simulink model "entreg2"  (R2019a)
settings: Solver=ode4  StartTime=0.0  StopTime=148  FixedStep=0.04  RelTol=1e-3
undefined symbols (not defined in the file or in its folder): Angular, Linear
libraries: robotlib x4, simulink x2, fuzblock x1
settings Model: Creator=LMI-01  LastModifiedBy=lucas
settings DataIOCC: ReturnWorkspaceOutputs=off
settings DebuggingCC: PregeneratedLibrarySubsystemCodeDiagnostic=none  ArithmeticOperatorsInVariantConditions=warning
settings SFSimCC: SimUseLocalCustomCode=off
settings RTWCC: RTWUseLocalCustomCode=off

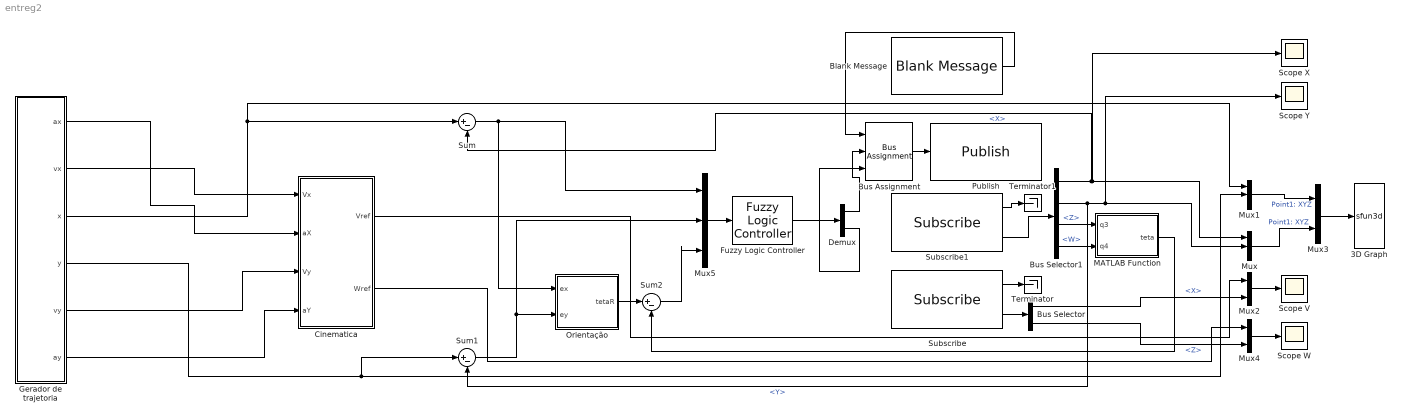
== system entreg2 ==
  3D Graph : S-Function  LoadFcn=if exist('sfun3d','file'), sfun3d([],[],[],'LoadBlock'); end  FunctionName=sfun3d  Parameters=ax,T,np,cp,gd,ls,mk,mx,hd,tb  SFunctionDeploymentMode=off  EnableBusSupport=off  mask(3D Graph){np=2, ax=[-6 6 -6 6 -3 3], mx=1e4, T=0.04, cp=[0 0 1], gd=on, hd=off, tb=on, ls=-, mk=none}
      mask prompts: np "Number of moving points (lines)"; ax "Range: [xmin xmax  ymin ymax zmin zmax]"; mx "Max number of points in each line"; T "Sampling Time"; cp "Camera position (use [0 0 1] for 2D XY view)"; gd "Grid (on|off)"; hd "HeadMarkers (on|off)"; tb "Toolbar (on|off)"; ls "LineStyle"; mk "LineMarker"
      mask help:
      | This block plots the position of several points in the XYZ space. The input contains the coordinates of all the points (x1,y1,z1,x2,y2,z2,...).
      | The number of moving points (lines), the XYZ ranges, sampling time, camera position, and grid (among other things) can be set as mask parameters.
      settings: CopyFcn=if exist('sfun3d','file'), sfun3d([],[],[],'CopyBlock'); end  DeleteFcn=if exist('sfun3d','file'), sfun3d([],[],[],'DeleteBlock'); end  NameChangeFcn=if exist('sfun3d','file'), sfun3d([],[],[],'NameChange'); end
      mask Help:
      | This block plots the position of several points in the XYZ space. The input contains the coordinates of all the points (x1,y1,z1,x2,y2,z2,...).
      | The number of moving points (lines), the XYZ ranges, sampling time, camera position, and grid (among other things) can be set as mask parameters.
      mask TypeOptions ls: - | -- | : | -. | none
      mask TypeOptions mk: none | . | + | o | * | x | square | diamond | v | ^ | > | < | pentagram | hexagram
      mask Display: plot([.05 .95 .95 .05 .05],[.45 .45 .95 .95 .45], 0.5+cos(0:0.1:2*pi)*0.3,0.7+sin(0:0.1:2*pi)*0.2)
  Blank Message : robotlib/Blank Message  messageClass=Message  entityType=geometry_msgs/Twist  messageType=geometry_msgs/Twist  SampleTime=inf
      settings: SourceProductBaseCode=RO
  Bus Assignment : BusAssignment  AssignedSignals=Linear.X,Angular.Z
  Bus Selector : BusSelector  OutputSignals=Linear.X,Angular.Z
  Bus Selector1 : BusSelector  OutputSignals=Pose.Pose.Position.X,Pose.Pose.Position.Y,Pose.Pose.Orientation.Z,Pose.Pose.Orientation.W
  Cinematica : MATLAB Function  TreatAsAtomicUnit=on
  Demux : Demux  Outputs=2
  Fuzzy Logic Controller : fuzblock/Fuzzy Logic  Controller  FIS='controlador_fuzzy2.fis'  OutputSampleNumber=101  DataType=double  FuzzifiedInputs=off  RuleFiringStrengths=off  RuleOutputs=off  AggregatedOutputs=off  SimulateUsing=Interpreted execution  OutOfRangeInputValueMessage=warning  NoRuleFiredMessage=warning  EmptyOutputFuzzySetMessage=warning
  "Gerador de trajetoria " : Subsystem
  MATLAB Function : MATLAB Function  TreatAsAtomicUnit=on
  Mux : Mux  Inputs=3
  Mux1 : Mux  Inputs=3
  Mux2 : Mux  Inputs=2
  Mux3 : Mux  Inputs=2
  Mux4 : Mux  Inputs=2
  Mux5 : Mux  Inputs=3
  Orientação : MATLAB Function  TreatAsAtomicUnit=on
  Publish : robotlib/Publish  topicSource=Select from ROS network  topic=/mobile_base/commands/velocity  messageType=geometry_msgs/Twist  messageQueueLength=1
      settings: SourceProductBaseCode=RO
  Scope V : Scope
  Scope W : Scope
  Scope X : Scope
  Scope Y : Scope
  Subscribe : robotlib/Subscribe  topicSource=Select from ROS network  topic=/mobile_base/commands/velocity  messageType=geometry_msgs/Twist  sampleTime=-1  messageQueueLength=1
      settings: SourceProductBaseCode=RO
  Subscribe1 : robotlib/Subscribe  topicSource=Select from ROS network  topic=/odom  messageType=nav_msgs/Odometry  sampleTime=-1  messageQueueLength=1
      settings: SourceProductBaseCode=RO
  Sum : Sum  Inputs=|+-
  Sum1 : Sum  Inputs=|+-
  Sum2 : Sum  Inputs=|+-
  Terminator : Terminator
  Terminator1 : Terminator
  wires:
  Mux/1 -> Mux3/2  "Point1: XYZ"
  Mux1/1 -> Mux3/1  "Point1: XYZ"
  Mux3/1 -> 3D Graph/1
  Bus Assignment/1 -> Publish/1
  Subscribe1/1 -> Terminator1/1
  Subscribe/1 -> Terminator/1
  Subscribe1/2 -> Bus Selector1/1
  Subscribe/2 -> Bus Selector/1
  Mux2/1 -> Scope V/1
  Mux4/1 -> Scope W/1
  Bus Selector1/4 -> MATLAB Function/2(q4)  "<W>"
  Bus Selector1/3 -> MATLAB Function/1(q3)  "<Z>"
  Bus Selector1/1 -> Sum/2, Mux/1, Scope X/1  "<X>"
  Bus Selector1/2 -> Sum1/2, Mux/2, Scope Y/1  "<Y>"
  Bus Selector/2 -> Mux4/2  "<Z>"
  Bus Selector/1 -> Mux2/2  "<X>"
  "Gerador de trajetoria "/6(ay) -> Cinematica/4(aY)
  "Gerador de trajetoria "/1(ax) -> Cinematica/2(aX)
  Cinematica/1(Vref) -> Mux2/1
  Sum2/1 -> Mux5/3
  Orientação/1(tetaR) -> Sum2/1
  Fuzzy Logic Controller/1 -> Demux/1
  Sum/1 -> Orientação/1(ex), Mux5/1
  Sum1/1 -> Orientação/2(ey), Mux5/2
  MATLAB Function/1(teta) -> Sum2/2
  "Gerador de trajetoria "/2(vx) -> Cinematica/1(Vx)
  Demux/2 -> Bus Assignment/3
  Demux/1 -> Bus Assignment/2
  Cinematica/2(Wref) -> Mux4/1
  "Gerador de trajetoria "/5(vy) -> Cinematica/3(Vy)
  Mux5/1 -> Fuzzy Logic Controller/1
  Blank Message/1 -> Bus Assignment/1
  "Gerador de trajetoria "/3(x) -> Mux1/1, Sum/1
  "Gerador de trajetoria "/4(y) -> Mux1/2, Sum1/1

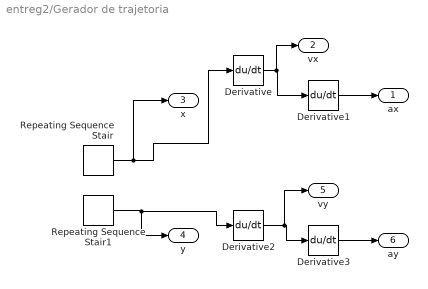
== system entreg2/Gerador de trajetoria  ==
  Derivative{,1..3} (4 alike) : Derivative
  Repeating Sequence Stair : simulink/Sources/Repeating Sequence Stair  OutValues=[0 0.35 0.7 1 1.17000000000000 1.13636630888818 1.29781681365468 1.46855831091587 1.63011117391398 1.86615524675713 2.01293235197162 2.16746647889735 2.18509923467053 2.19795065796801 2.19797948716949 2.22496970011073 2.24304671068726 2.23929618970334 2.26982794069553 2.26080362632337 2.38874656381839 2.50687255452925 2.60796600466398 2.75842470931807 2.91812309896753 3.09994531392603 3.21130779193203 3.37786059481534 3.37640575264878 3.45327720396131 3.47739985849164 3.52177306258873 3.57218392139281 3.68133849097106 3.84273878303952 3.97251349229218 4.19159254394481 4.39520776047253 4.72269852816546 5.06130600308634 5.36152509053121 5.59879385999157 5.61395180134724 5.57505150961989 5.56764716952759 5.51257506819779 5.51874953704695 5.50000000000000]  tsamp=3.20  OutMin=[]  OutMax=[]  OutDataTypeStr=double  OutputDataTypeScalingMode=double  OutDataType=fixdt(0,8)  ConRadixGroup=Best Precision: Vector-wise  OutScaling=2^-12
  Repeating Sequence Stair1 : simulink/Sources/Repeating Sequence Stair  OutValues=[-0.35 -0.35 -0.35 -0.35 0.0651893966525788 0.362129707732075 0.623753677382057 0.775354419626675 0.961745396579764 1.09086894927094 1.33822349520960 1.61879248910219 1.69784845568527 2.02858237206169 2.25979192143125 2.45253391279033 2.67050764424766 2.97554368142654 3.25003618292319 3.50994458764924 3.58083763030385 3.60607486682255 3.63371834792494 3.62325351902815 3.57869462970668 3.52263302654614 3.23603577016277 2.97281325291245 2.66960102131579 2.50992729488802 2.16798337821201 1.84910828582459 1.64510890890260 1.46272820883164 1.23525461377249 0.982385103207933 0.878102802302353 0.892639115809230 0.881338079577862 0.868529585350037 1.10708558244037 1.37592837094794 1.68515277057135 1.96863003655324 2.28149720632578 2.48742341640947 2.50000000000000]  tsamp=3.20  OutMin=[]  OutMax=[]  OutDataTypeStr=double  OutputDataTypeScalingMode=double  OutDataType=fixdt(0,8)  ConRadixGroup=Best Precision: Vector-wise  OutScaling=2^-12
  ax : Outport
  vx : Outport  Port=2
  x : Outport  Port=3
  y : Outport  Port=4
  vy : Outport  Port=5
  ay : Outport  Port=6
  wires:
  Derivative1/1 -> ax/1
  Derivative/1 -> vx/1, Derivative1/1
  Repeating Sequence Stair1/1 -> Derivative2/1, y/1
  Repeating Sequence Stair/1 -> x/1, Derivative/1
  Derivative2/1 -> vy/1, Derivative3/1
  Derivative3/1 -> ay/1

== matlab function entreg2/MATLAB Function ==
  data: q3 input; teta output; q4 input
function teta = fcn2(q3,q4)
teta=2*atan2(q3,q4);

== matlab function entreg2/Orientação ==
  data: ex input; tetaR output; ey input
function tetaR  = fcn(ex, ey)

tetaR = atan2(ey,ex);

end

== matlab function entreg2/Cinematica ==
  data: Vx input; aX input; Vy input; aY input; Vref output; Wref output
function [Vref, Wref] = fcn(Vx, aX, Vy, aY)

Vref = sqrt(Vx^2 + Vy^2);
Wref = (Vx*aY - Vy*aX)/(Vx^2 + Vy^2);

end
